simulink model "ESM_mdl"  (R2024b)
settings: Solver=ode4  StartTime=0.0  StopTime=tdur  FixedStep=dt_sim  RelTol=1e-10
values from neighbouring files (symbols this model uses):
  alpha_dem = 0    [ESM_harness.m]    (also in ESM_mat.mat)
  beta_dem = 0    [ESM_harness.m]    (also in ESM_mat.mat)
  dt_sim = 0.1    [ESM_harness.m]    (also in ESM_mat.mat)
  Kdx = 5000    [ESM_harness.m]    (also in ESM_mat.mat)
  Kdy = 15000    [ESM_harness.m]    (also in ESM_mat.mat)
  Kdz = 1700    [ESM_harness.m]    (also in ESM_mat.mat)
  Kpx = 125    [ESM_harness.m]    (also in ESM_mat.mat)
  Kpy = 375    [ESM_harness.m]    (also in ESM_mat.mat)
  Krcs = 1    [ESM_harness.m]    (also in ESM_mat.mat)
  rate_sensor_model_type = 2    [ESM_harness.m]    (also in ESM_mat.mat)
  s_i = [0 0 1]'    [ESM_harness.m]    (also in ESM_mat.mat = [0 0 1])
  sigma_w = 0.0005/r2d    (= 8.72664625997e-06)    [ESM_harness.m]    (also in ESM_mat.mat)
  T_env = [0.1 0.1 0.1]'    [ESM_harness.m]    (also in ESM_mat.mat = [0.1 0.1 0.1])
  ta = 0.5    [ESM_harness.m]    (also in ESM_mat.mat)
  tdelay = 0.2    [ESM_harness.m]    (also in ESM_mat.mat)
  w_bias = [0 0 -0.1]/r2d    [ESM_harness.m]    (also in ESM_mat.mat = [0 0 -0.00174532925199])
libraries: spacecraft_simulink_library x6
settings Model: Creator=HARDAC_S  LastModifiedBy=Rich
settings SolverCC: AlgebraicLoopSolver=TrustRegion
settings DataIOCC: SaveFormat=Array  SignalLoggingSaveFormat=ModelDataLogs  SaveOutput=off  ReturnWorkspaceOutputs=off  SignalLoggingName=sigsOut
settings OptimizationCC: ExpressionDepthLimit=2147483647  InitFltsAndDblsToZero=on  LifeSpan=inf
settings DebuggingCC: SaveWithParameterizedLinksMsg=none  UnderspecifiedInitializationDetection=Classic  MergeDetectMultiDrivingBlocksExec=none  SignalResolutionControl=TryResolveAllWithWarning  MultiTaskDSMMsg=warning  MultiTaskCondExecSysMsg=none  FcnCallInpInsideContextMsg=warning  UnconnectedInputMsg=warning  UnconnectedOutputMsg=warning  UnconnectedLineMsg=warning  AllowSymbolicDim=off  StateNameClashWarn=warning  SFUnexpectedBacktrackingDiag=warning  SFNoUnconditionalDefaultTransitionDiag=warning  SFExecutionAtInitializationDiag=none  ArithmeticOperatorsInVariantConditions=warning
settings HardwareCC: ProdBitPerPointer=32  ProdBitPerSizeT=32  ProdBitPerPtrDiffT=32  ProdLargestAtomicFloat=None  ProdIntDivRoundTo=Undefined  ProdEndianess=Unspecified  ProdWordSize=32  ProdHWDeviceType=32-bit Generic  TargetUnknown=on
settings ModelReferenceCC: EnableRefExpFcnMdlSchedulingChecks=on  PropagateSignalLabelsOutOfModel=off
settings SFSimCC: SimUseLocalCustomCode=off  SimParseCustomCode=off  CustomCodeUndefinedFunction=UseInterfaceOnly
settings RTWCC: RTWUseLocalCustomCode=off  GPUComputeCapability=3.5
settings CodeAppCC: StateflowObjectComments=on
settings GRTTargetCC: TargetLangStandard=C89/C90 (ANSI)  CombineOutputUpdateFcns=off  GRTInterface=on
settings ConfigComp: CovMetricSettings=dw  CovSaveCumulativeToWorkspaceVar=on  CovSaveSingleToWorkspaceVar=on  CovExternalEMLEnable=off

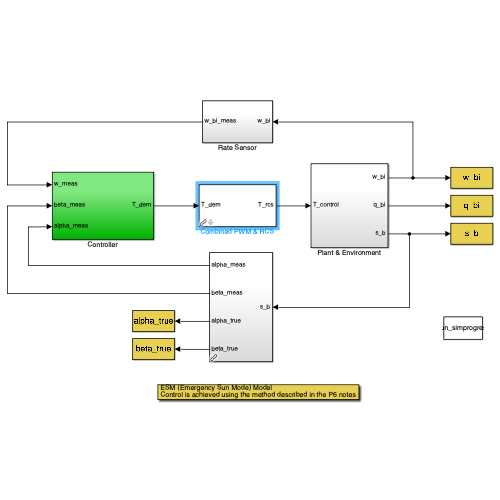
[thumbnail: Simulink's stored preview of the top-level diagram]
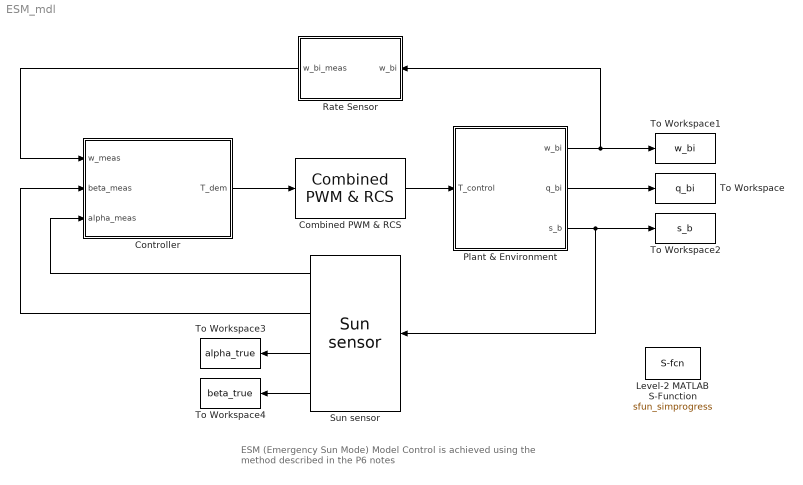
== system ESM_mdl ==
  note: ESM (Emergency Sun Mode) Model
      | Control is achieved using the method described in the P6 notes
  Combined PWM & RCS : spacecraft_simulink_library/Combined PWM & RCS  T_deadband=Tdb  T_saturation=Trcs_saturation  K_rcs=[Krcs Krcs Krcs]
  Controller : Subsystem
  Level-2 MATLAB S-Function : M-S-Function  FunctionName=sfun_simprogress  Parameters=100
  Plant & Environment : Subsystem
  Rate Sensor : Subsystem
  Sun sensor : spacecraft_simulink_library/Sun sensor  SystemSampleTime=-1  VariantActivationTime=update diagram  AllowFlexibleInterface=on  Latency=0  AutoFrameSizeCalculation=off
  To Workspace : ToWorkspace  VariableName=q_bi  SampleTime=-1
  To Workspace1 : ToWorkspace  VariableName=w_bi  SampleTime=-1
  To Workspace2 : ToWorkspace  VariableName=s_b  SampleTime=-1
  To Workspace3 : ToWorkspace  VariableName=alpha_true  SampleTime=-1
  To Workspace4 : ToWorkspace  VariableName=beta_true  SampleTime=-1
  wires:
  Controller/1(T_dem) -> Combined PWM & RCS/1
  Plant & Environment/1(w_bi) -> Rate Sensor/1(w_bi), To Workspace1/1
  Plant & Environment/3(s_b) -> To Workspace2/1, Sun sensor/1
  Plant & Environment/2(q_bi) -> To Workspace/1
  Sun sensor/1 -> Controller/3(alpha_meas)
  Rate Sensor/1(w_bi_meas) -> Controller/1(w_meas)
  Sun sensor/2 -> Controller/2(beta_meas)
  Combined PWM & RCS/1 -> Plant & Environment/1(T_control)
  Sun sensor/3 -> To Workspace3/1
  Sun sensor/4 -> To Workspace4/1

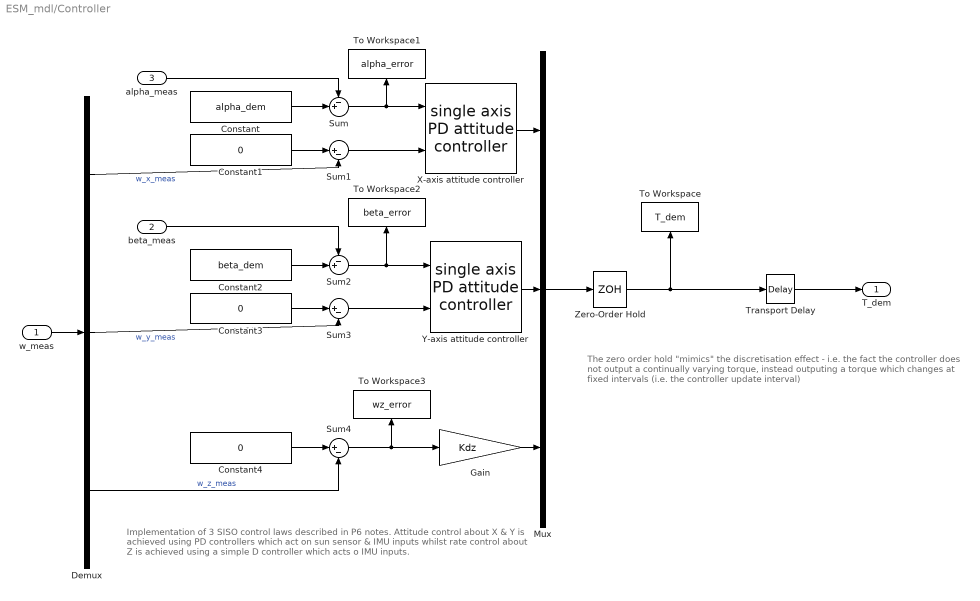
== system ESM_mdl/Controller ==
  note: The zero order hold "mimics" the discretisation effect - i.e. the fact the controller
      | does not output a continually varying torque, instead outputing a torque which
      | changes at fixed intervals (i.e. the controller update interval)
  note: Implementation of 3 SISO control laws described in P6 notes. Attitude control about
      | X & Y is achieved using PD controllers which act on sun sensor & IMU inputs whilst rate
      | control about Z is achieved using a simple D controller which acts o IMU inputs.
  w_meas : Inport
  beta_meas : Inport  Port=2
  alpha_meas : Inport  Port=3
  Constant : Constant  Value=alpha_dem
  Constant1 : Constant  Value=0
  Constant2 : Constant  Value=beta_dem
  Constant3 : Constant  Value=0
  Constant4 : Constant  Value=0
  Demux : Demux  Outputs=3
      settings: DisplayOption=none
  Gain : Gain  Gain=Kdz  SaturateOnIntegerOverflow=on  OutDataTypeStr=Inherit: Same as input  ParamDataTypeStr=Inherit: Same as input
  Mux : Mux  Inputs=3
  Sum : Sum  Inputs=-+|  SaturateOnIntegerOverflow=on
  Sum1 : Sum  Inputs=|+-  SaturateOnIntegerOverflow=on
  Sum2 : Sum  Inputs=-+|  SaturateOnIntegerOverflow=on
  Sum3 : Sum  Inputs=|+-  SaturateOnIntegerOverflow=on
  Sum4 : Sum  Inputs=|+-  SaturateOnIntegerOverflow=on
  To Workspace : ToWorkspace  VariableName=T_dem  SampleTime=dt_sim
  To Workspace1 : ToWorkspace  VariableName=alpha_error  SampleTime=dt_sim
  To Workspace2 : ToWorkspace  VariableName=beta_error  SampleTime=dt_sim
  To Workspace3 : ToWorkspace  VariableName=wz_error  SampleTime=dt_sim
  Transport Delay : TransportDelay  DelayTime=tdelay
  X-axis attitude controller : spacecraft_simulink_library/single axis PD attitude controller  Kp=Kpx  Kd=Kdx
  Y-axis attitude controller : spacecraft_simulink_library/single axis PD attitude controller  Kp=Kpy  Kd=Kdy
  Zero-Order Hold : ZeroOrderHold  SampleTime=ta
  T_dem : Outport
  wires:
  Sum/1 -> X-axis attitude controller/1, To Workspace1/1
  Constant1/1 -> Sum1/1
  Sum1/1 -> X-axis attitude controller/2
  Constant/1 -> Sum/2
  Sum2/1 -> Y-axis attitude controller/1, To Workspace2/1
  Constant3/1 -> Sum3/1
  Sum3/1 -> Y-axis attitude controller/2
  Constant2/1 -> Sum2/2
  alpha_meas/1 -> Sum/1
  X-axis attitude controller/1 -> Mux/1
  Demux/1 -> Sum1/2  "w_x_meas"
  Y-axis attitude controller/1 -> Mux/2
  Demux/2 -> Sum3/2  "w_y_meas"
  Mux/1 -> Zero-Order Hold/1
  w_meas/1 -> Demux/1
  beta_meas/1 -> Sum2/1
  Gain/1 -> Mux/3
  Demux/3 -> Sum4/2  "w_z_meas"
  Sum4/1 -> Gain/1, To Workspace3/1
  Constant4/1 -> Sum4/1
  Zero-Order Hold/1 -> To Workspace/1, Transport Delay/1
  Transport Delay/1 -> T_dem/1

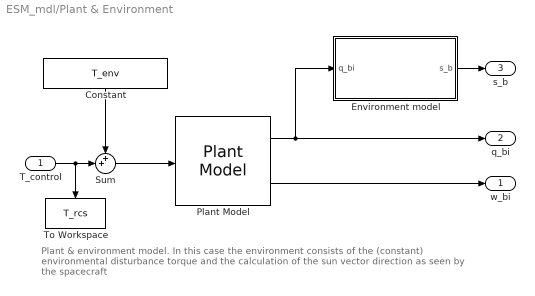
== system ESM_mdl/Plant & Environment ==
  note: Plant & environment model.
      |
      | In this case the environment consists of the (constant) environmental disturbance torque
      | and the calculation of the sun vector direction as seen by the spacecraft
  T_control : Inport
  Constant : Constant  Value=T_env
  Environment model : Subsystem
      mask Display: disp('determine sun vector\nin body frame')
  Plant Model : spacecraft_simulink_library/Plant Model  SystemSampleTime=-1  VariantActivationTime=update diagram  AllowFlexibleInterface=on  Latency=0  AutoFrameSizeCalculation=off
  Sum : Sum  Inputs=++|  SaturateOnIntegerOverflow=on
  To Workspace : ToWorkspace  VariableName=T_rcs  SampleTime=dt_sim
  w_bi : Outport
  q_bi : Outport  Port=2
  s_b : Outport  Port=3
  wires:
  Plant Model/1 -> Environment model/1(q_bi), q_bi/1
  Plant Model/2 -> w_bi/1
  Environment model/1(s_b) -> s_b/1
  T_control/1 -> Sum/2, To Workspace/1
  Sum/1 -> Plant Model/1
  Constant/1 -> Sum/1

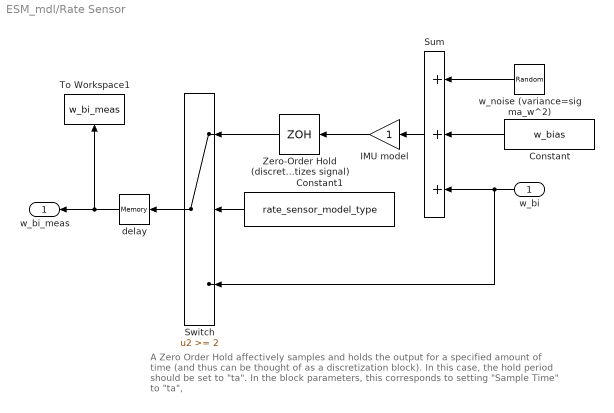
== system ESM_mdl/Rate Sensor ==
  note: A Zero Order Hold affectively samples and holds the output for a specified amount
      | of time (and thus can be thought of as a discretization block). In this case, the hold
      | period should be set to "ta". In the block parameters, this corresponds to setting
      | "Sample Time" to "ta",
  w_bi : Inport
  Constant : Constant  Value=w_bias
  Constant1 : Constant  Value=rate_sensor_model_type
  IMU model : Gain  SaturateOnIntegerOverflow=on  OutDataTypeStr=Inherit: Same as input  ParamDataTypeStr=Inherit: Same as input
  Sum : Sum  Inputs=+++  SaturateOnIntegerOverflow=on
  Switch : Switch  Threshold=2  InputSameDT=off
  To Workspace1 : ToWorkspace  VariableName=w_bi_meas  SampleTime=dt_sim
  Zero-Order Hold (discretetizes signal) : ZeroOrderHold  SampleTime=ta
  delay : Memory
  w_noise (variance=sigma_w^2) : RandomNumber  Variance=sigma_w^2  SampleTime=0
  w_bi_meas : Outport
  wires:
  IMU model/1 -> Zero-Order Hold (discretetizes signal)/1
  w_noise (variance=sigma_w^2)/1 -> Sum/1
  Sum/1 -> IMU model/1
  Constant/1 -> Sum/2
  w_bi/1 -> Sum/3, Switch/3
  Zero-Order Hold (discretetizes signal)/1 -> Switch/1
  Switch/1 -> delay/1
  Constant1/1 -> Switch/2
  delay/1 -> w_bi_meas/1, To Workspace1/1

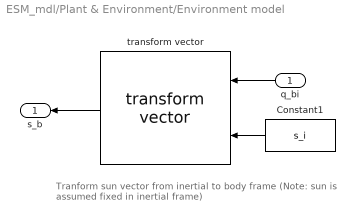
== system ESM_mdl/Plant & Environment/Environment model ==
  note: Tranform sun vector from inertial to body frame (Note: sun is
      | assumed fixed in inertial frame)
  q_bi : Inport
  Constant1 : Constant  Value=s_i
  transform vector : spacecraft_simulink_library/transform vector  SystemSampleTime=-1  VariantActivationTime=update diagram  AllowFlexibleInterface=on  Latency=0  AutoFrameSizeCalculation=off
  s_b : Outport
  wires:
  q_bi/1 -> transform vector/1
  Constant1/1 -> transform vector/2
  transform vector/1 -> s_b/1
